simulink model "basic_dynamic_ant"  (R2022a)
settings: Solver=VariableStepAuto  StartTime=0.0  StopTime=10.0  RelTol=1e-3
values from neighbouring files (symbols this model uses):
  configSequence = [robot.Bodies{4}.Joint.PositionLimits; -robot.Bodies{7}.Joint.PositionLimits]    [ant_grasp_only.m]
  dq0 = zeros(size(q0))    [ant_grasp_only.m]
  q0 = homeConfiguration(robot)    [ant_grasp_only.m]
  widgetDimensions = [0.2 0.02 0.07]    [ant_grasp_only.m]
undefined symbols (not defined in the file or in its folder): CenterTable, Floor, LeftShelf, X, Y, Z
libraries: sm_lib x137, nesl_utility x13, robotmaniplib x3, robotcorelib x1
(part 1 of 5)
settings Model: Creator=eroll  LastModifiedBy=eroll

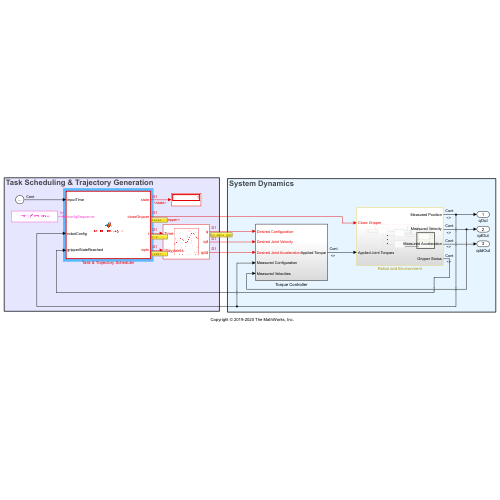
[thumbnail: Simulink's stored preview of the top-level diagram]
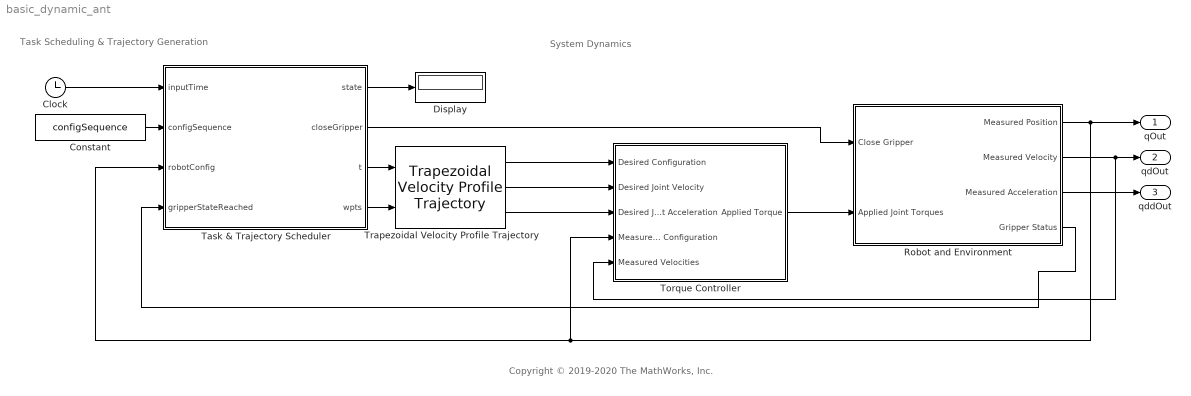
== system basic_dynamic_ant ==
  note: System Dynamics
  note: Copyright © 2019-2020 The MathWorks, Inc.
  note: Task Scheduling & Trajectory Generation
  Clock : Clock
  Constant : Constant  Value=configSequence
  Display : Display
  Robot and Environment : Subsystem
  Task & Trajectory Scheduler : MATLAB Function  TreatAsAtomicUnit=on
  Torque Controller : Subsystem
  Trapezoidal Velocity Profile Trajectory : robotcorelib/Trapezoidal Velocity Profile Trajectory  WaypointSource=External  Waypoints=[ 0, -0.5, -1; 0, 0.5, 1 ]  NumParams=1  Parameter1=End Time  Parameter2=End Time  ParameterSource=Internal  PeakVelocity=[ 2; 2 ]  Acceleration=[ 1; 2 ]  EndTime=2  AccelTime=[ 1; 2 ]  SimulateUsing=Interpreted execution
      settings: SourceProductBaseCode=RO,NV,RR,UV
  qOut : Outport
  qdOut : Outport  Port=2
  qddOut : Outport  Port=3
  wires:
  Task & Trajectory Scheduler/1(state) -> Display/1
  Robot and Environment/4(Gripper Status) -> Task & Trajectory Scheduler/4(gripperStateReached)
  Trapezoidal Velocity Profile Trajectory/1 -> Torque Controller/1(Desired Configuration)
  Clock/1 -> Task & Trajectory Scheduler/1(inputTime)
  Trapezoidal Velocity Profile Trajectory/3 -> Torque Controller/3(Desired Joint Acceleration)
  Trapezoidal Velocity Profile Trajectory/2 -> Torque Controller/2(Desired Joint Velocity)
  Task & Trajectory Scheduler/3(t) -> Trapezoidal Velocity Profile Trajectory/1
  Task & Trajectory Scheduler/4(wpts) -> Trapezoidal Velocity Profile Trajectory/2
  Constant/1 -> Task & Trajectory Scheduler/2(configSequence)
  Task & Trajectory Scheduler/2(closeGripper) -> Robot and Environment/1(Close Gripper)
  Robot and Environment/1(Measured Position) -> Torque Controller/4(Measured Configuration), Task & Trajectory Scheduler/3(robotConfig), qOut/1
  Torque Controller/1(Applied Torque) -> Robot and Environment/2(Applied Joint Torques)
  Robot and Environment/2(Measured Velocity) -> Torque Controller/5(Measured Velocities), qdOut/1
  Robot and Environment/3(Measured Acceleration) -> qddOut/1

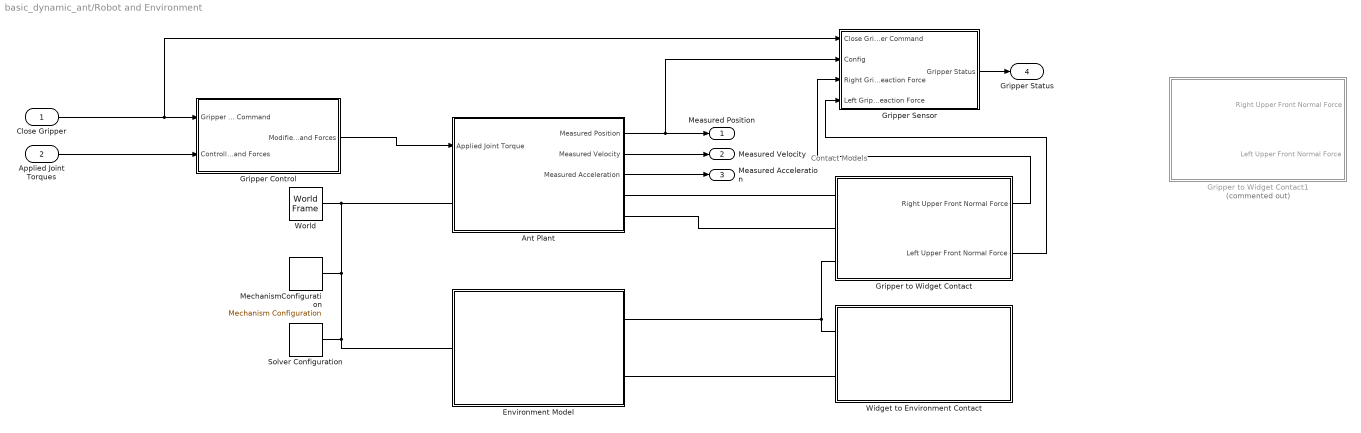
== system basic_dynamic_ant/Robot and Environment ==
  note: Contact Models
  Close Gripper : Inport
  Applied Joint Torques : Inport  Port=2
  Ant Plant : Subsystem
  Environment Model : Subsystem
  Gripper Control : Subsystem
  Gripper Sensor : Subsystem
  Gripper to Widget Contact : Subsystem
  Gripper to Widget Contact1 : Subsystem  Commented=on
  MechanismConfiguration : sm_lib/Utilities/Mechanism Configuration  UniformGravity=Constant  GravityVector=[0 0 -9.80665]  GravityUnits=m/s^2  LinearizationDelta=0.001  JointModeTransitionNonlinearIterations=2
  Solver Configuration : nesl_utility/Solver Configuration  PhysicalDomain=network_engine_domain  SubClassName=solver  LeftPortType=input  RightPortType=generic  Tones=[]  Harmonics=[]  SimulateNoise=off  Profile=off  UseLocalSampling=off  EnableSwitchedLinearOptims=on  FrequencyDomain=off  UseCCode=off  RelTol=0.001  AbsTol=1e-06  MinStep=1e-09  ToWorkspace=off  RevertToSquareIcSolve=off  NumHomotopyIterations=100  PhasorMode=off  PhasorModeNumHarmonics=1  IndexReductionMethod=DerivativeReplacement  DoDC=off  ResidualTolerance=1e-09  UseLocalSolver=off  LocalSolverChoice=NE_BACKWARD_EULER_ADVANCER  LocalSolverSampleTime=0.001  DoFixedCost=off  MaxNonlinIter=3  MaxModeIter=2  ComputeImpulses=off  ImpulseIterations=2  LinearAlgebra=auto  LinearAlgebraNumThread=0  EquationFormulation=NE_TIME_EF  DelaysMemoryBudget=1024  AutomaticFiltering=on  FilteringTimeConstant=0.001  PartitionStorageMethod=AS_NEEDED  PartitionMemoryBudget=1024  PartitionMethod=ROBUST
      settings: SourceProductBaseCode=SS,PW,VE
  Widget to Environment Contact : Subsystem
  World : sm_lib/Frames and Transforms/World Frame
  Measured Position : Outport
  Measured Velocity : Outport  Port=2
  Measured Acceleration : Outport  Port=3
  Gripper Status : Outport  Port=4
  wires:
  Ant Plant/2(Measured Velocity) -> Measured Velocity/1
  Ant Plant/3(Measured Acceleration) -> Measured Acceleration/1
  Applied Joint Torques/1 -> Gripper Control/2(Controller Joint Torques and Forces)
  Gripper Control/1(Modified Joint Torques and Forces) -> Ant Plant/1(Applied Joint Torque)
  Close Gripper/1 -> Gripper Sensor/1(Close Gripper Command), Gripper Control/1(Gripper Close Command)
  Gripper to Widget Contact/1(Right Upper Front Normal Force) -> Gripper Sensor/3(Right Gripper Reaction Force)
  Gripper Sensor/1(Gripper Status) -> Gripper Status/1
  Ant Plant/1(Measured Position) -> Gripper Sensor/2(Config), Measured Position/1
  Gripper to Widget Contact/2(Left Upper Front Normal Force) -> Gripper Sensor/4(Left Gripper Reaction Force)
  connections:
  World/RConn1 -- Ant Plant/LConn1 -- Environment Model/LConn1 -- Solver Configuration/RConn1 -- MechanismConfiguration/RConn1
  Widget to Environment Contact/LConn1 -- Gripper to Widget Contact/LConn3 -- Environment Model/RConn1
  Environment Model/RConn2 -- Widget to Environment Contact/LConn2
  Ant Plant/RConn2 -- Gripper to Widget Contact/LConn2
  Ant Plant/RConn1 -- Gripper to Widget Contact/LConn1

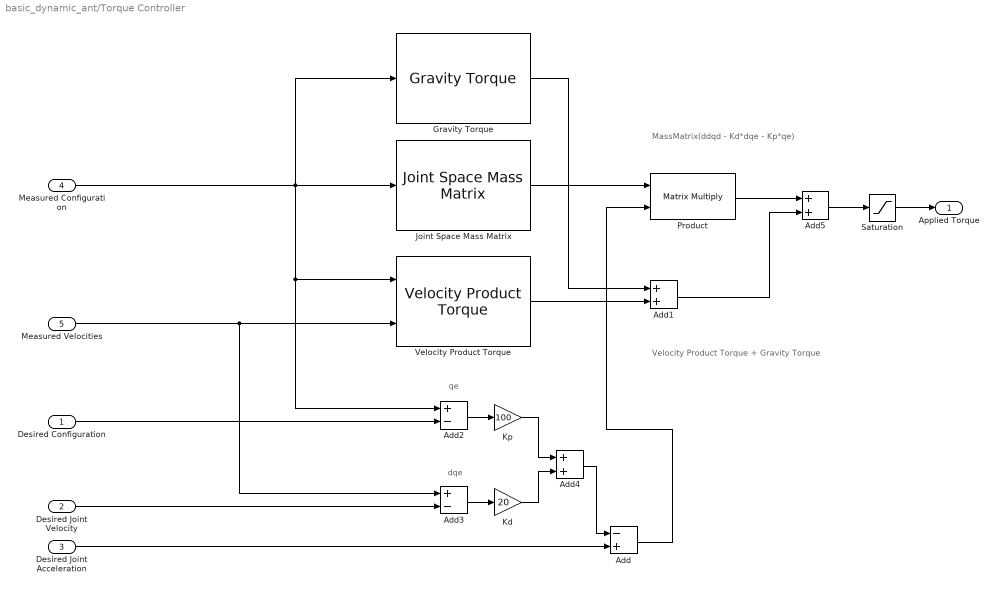
== system basic_dynamic_ant/Torque Controller ==
  note: qe
  note: dqe
  note: Velocity Product Torque + Gravity Torque
  note: MassMatrix(ddqd - Kd*dqe - Kp*qe)
  Desired Configuration : Inport
  Desired Joint Velocity : Inport  Port=2
  Desired Joint Acceleration : Inport  Port=3
  Measured Configuration : Inport  Port=4
  Measured Velocities : Inport  Port=5
  Add : Sum  Inputs=-+
  Add1 : Sum
  Add2 : Sum  Inputs=+-
  Add3 : Sum  Inputs=+-
  Add4 : Sum
  Add5 : Sum
  Gravity Torque : robotmaniplib/Gravity Torque  RigidBodyTree=robot  SimulateUsing=Interpreted execution
  Joint Space Mass Matrix : robotmaniplib/Joint Space Mass Matrix  RigidBodyTree=robot  SimulateUsing=Interpreted execution
  Kd : Gain  Gain=20
  Kp : Gain  Gain=100
  Product : Product  Multiplication=Matrix(*)
  Saturation : Saturate  UpperLimit=100  LowerLimit=-100
  Velocity Product Torque : robotmaniplib/Velocity Product Torque  RigidBodyTree=robot  SimulateUsing=Interpreted execution
      settings: SourceProductBaseCode=RO
  Applied Torque : Outport  VectorParamsAs1DForOutWhenUnconnected=off
  wires:
  Desired Joint Acceleration/1 -> Add/2
  Desired Joint Velocity/1 -> Add3/2
  Desired Configuration/1 -> Add2/2
  Joint Space Mass Matrix/1 -> Product/1
  Measured Configuration/1 -> Joint Space Mass Matrix/1, Gravity Torque/1, Velocity Product Torque/1, Add2/1
  Measured Velocities/1 -> Add3/1, Velocity Product Torque/2
  Add4/1 -> Add/1
  Add/1 -> Product/2
  Add2/1 -> Kp/1
  Add3/1 -> Kd/1
  Kp/1 -> Add4/1
  Kd/1 -> Add4/2
  Add5/1 -> Saturation/1
  Product/1 -> Add5/1
  Add1/1 -> Add5/2
  Gravity Torque/1 -> Add1/1
  Velocity Product Torque/1 -> Add1/2
  Saturation/1 -> Applied Torque/1

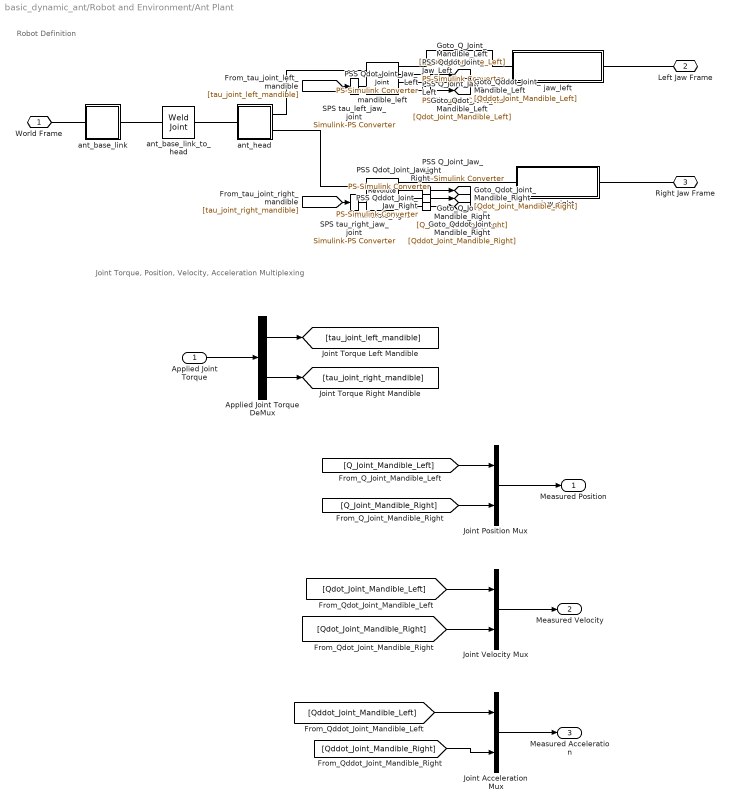
== system basic_dynamic_ant/Robot and Environment/Ant Plant ==
  note: Robot Definition
  note: Joint Torque, Position, Velocity, Acceleration Multiplexing
  Applied Joint Torque : Inport
  Applied Joint Torque DeMux : Demux  Outputs=2
  Joint Acceleration Mux : Mux  Inputs=2
  Joint Position Mux : Mux  Inputs=2
  Joint Velocity Mux : Mux  Inputs=2
  PSS Q_Joint_Jaw_Left : nesl_utility/PS-Simulink Converter  PhysicalDomain=network_engine_domain  SubClassName=ps_output  LeftPortType=input  RightPortType=output  PseudoPeriodic=off  Frequencies=[]  VectorFormat=1-D array  Unit=inherit  AffineConversion=off
      settings: SourceProductBaseCode=SS,PW,VE
  PSS Q_Joint_Jaw_Right : nesl_utility/PS-Simulink Converter  PhysicalDomain=network_engine_domain  SubClassName=ps_output  LeftPortType=input  RightPortType=output  PseudoPeriodic=off  Frequencies=[]  VectorFormat=1-D array  Unit=inherit  AffineConversion=off
      settings: SourceProductBaseCode=SS,PW,VE
  PSS Qddot_Joint_Jaw_Left : nesl_utility/PS-Simulink Converter  PhysicalDomain=network_engine_domain  SubClassName=ps_output  LeftPortType=input  RightPortType=output  PseudoPeriodic=off  Frequencies=[]  VectorFormat=1-D array  Unit=inherit  AffineConversion=off
      settings: SourceProductBaseCode=SS,PW,VE
  PSS Qddot_Joint_Jaw_Right : nesl_utility/PS-Simulink Converter  PhysicalDomain=network_engine_domain  SubClassName=ps_output  LeftPortType=input  RightPortType=output  PseudoPeriodic=off  Frequencies=[]  VectorFormat=1-D array  Unit=inherit  AffineConversion=off
      settings: SourceProductBaseCode=SS,PW,VE
  PSS Qdot_Joint_Jaw_Left : nesl_utility/PS-Simulink Converter  PhysicalDomain=network_engine_domain  SubClassName=ps_output  LeftPortType=input  RightPortType=output  PseudoPeriodic=off  Frequencies=[]  VectorFormat=1-D array  Unit=inherit  AffineConversion=off
      settings: SourceProductBaseCode=SS,PW,VE
  PSS Qdot_Joint_Jaw_Right : nesl_utility/PS-Simulink Converter  PhysicalDomain=network_engine_domain  SubClassName=ps_output  LeftPortType=input  RightPortType=output  PseudoPeriodic=off  Frequencies=[]  VectorFormat=1-D array  Unit=inherit  AffineConversion=off
      settings: SourceProductBaseCode=SS,PW,VE
  SPS tau_left_jaw_joint : nesl_utility/Simulink-PS Converter  PhysicalDomain=network_engine_domain  SubClassName=ps_input  LeftPortType=input  RightPortType=output  PseudoPeriodic=off  Frequencies=[]  NoiseDistribution=none  NoiseParameters=[]  Unit=1  AffineConversion=off  FilteringAndDerivatives=provide  SimscapeFilterOrder=1  InputFilterTimeConstant=0.001  UdotUserProvided=0
      settings: SourceProductBaseCode=SS,PW,VE
  SPS tau_right_jaw_joint : nesl_utility/Simulink-PS Converter  PhysicalDomain=network_engine_domain  SubClassName=ps_input  LeftPortType=input  RightPortType=output  PseudoPeriodic=off  Frequencies=[]  NoiseDistribution=none  NoiseParameters=[]  Unit=1  AffineConversion=off  FilteringAndDerivatives=provide  SimscapeFilterOrder=1  InputFilterTimeConstant=0.001  UdotUserProvided=0
      settings: SourceProductBaseCode=SS,PW,VE
  ant_base_link : Subsystem
  ant_base_link_to_head : sm_lib/Joints/Weld Joint  JointMode=Normal  SenseConstraintForce=off  SenseConstraintForceX=off  SenseConstraintForceY=off  SenseConstraintForceZ=off  SenseConstraintTorque=off  SenseConstraintTorqueX=off  SenseConstraintTorqueY=off  SenseConstraintTorqueZ=off  SenseTotalForce=off  SenseTotalForceX=off  SenseTotalForceY=off  SenseTotalForceZ=off  SenseTotalTorque=off  SenseTotalTorqueX=off  SenseTotalTorqueY=off  SenseTotalTorqueZ=off  CompositeWrenchDir=FollowerOnBase  CompositeWrenchFrame=BaseFrame
  ant_head : Subsystem
  jaw_left : Subsystem
  jaw_right : Subsystem
  mandible_left : sm_lib/Joints/Revolute Joint  JointMode=Normal  SenseConstraintForce=off  SenseConstraintForceX=off  SenseConstraintForceY=off  SenseConstraintForceZ=off  SenseConstraintTorque=off  SenseConstraintTorqueX=off  SenseConstraintTorqueY=off  SenseConstraintTorqueZ=off  SenseTotalForce=off  SenseTotalForceX=off  SenseTotalForceY=off  SenseTotalForceZ=off  SenseTotalTorque=off  SenseTotalTorqueX=off  SenseTotalTorqueY=off  SenseTotalTorqueZ=off  CompositeWrenchDir=FollowerOnBase  CompositeWrenchFrame=BaseFrame  EquilibriumPosition=0  EquilibriumPositionUnits=deg  SpringStiffness=0  SpringStiffnessUnits=N*m/deg  DampingCoefficient=0.5  DampingCoefficientUnits=m^2*kg/s/rad  TorqueActuationMode=InputTorque  MotionActuationMode=ComputedMotion  SensePosition=on  SenseVelocity=on  SenseAcceleration=on  SenseTorqueForce=off  SenseLowerLimitTorqueForce=off  SenseUpperLimitTorqueForce=off  LowerLimitSpecify=on  LowerLimitBound=-2.94087978961  LowerLimitBoundUnits=rad  LowerLimitStiffness=1e4  LowerLimitStiffnessUnits=N*m/deg  LowerLimitDamping=10  LowerLimitDampingUnits=N*m/(deg/s)  LowerLimitTransitionRegionWidth=0.1  LowerLimitTransitionRegionWidthUnits=deg  UpperLimitSpecify=on  UpperLimitBound=2.94087978961  UpperLimitBoundUnits=rad  UpperLimitStiffness=1e4  UpperLimitStiffnessUnits=N*m/deg  UpperLimitDamping=10  UpperLimitDampingUnits=N*m/(deg/s)  UpperLimitTransitionRegionWidth=0.1  UpperLimitTransitionRegionWidthUnits=deg  PositionTargetSpecify=on  PositionTargetPriority=High  PositionTargetValue=q0(1)  PositionTargetValueUnits=rad  VelocityTargetSpecify=on  VelocityTargetPriority=High  VelocityTargetValue=dq0(1)  VelocityTargetValueUnits=rad/s
  mandible_right : sm_lib/Joints/Revolute Joint  JointMode=Normal  SenseConstraintForce=off  SenseConstraintForceX=off  SenseConstraintForceY=off  SenseConstraintForceZ=off  SenseConstraintTorque=off  SenseConstraintTorqueX=off  SenseConstraintTorqueY=off  SenseConstraintTorqueZ=off  SenseTotalForce=off  SenseTotalForceX=off  SenseTotalForceY=off  SenseTotalForceZ=off  SenseTotalTorque=off  SenseTotalTorqueX=off  SenseTotalTorqueY=off  SenseTotalTorqueZ=off  CompositeWrenchDir=FollowerOnBase  CompositeWrenchFrame=BaseFrame  EquilibriumPosition=0  EquilibriumPositionUnits=deg  SpringStiffness=0  SpringStiffnessUnits=N*m/deg  DampingCoefficient=0.5  DampingCoefficientUnits=m^2*kg/s/rad  TorqueActuationMode=InputTorque  MotionActuationMode=ComputedMotion  SensePosition=on  SenseVelocity=on  SenseAcceleration=on  SenseTorqueForce=off  SenseLowerLimitTorqueForce=off  SenseUpperLimitTorqueForce=off  LowerLimitSpecify=off  LowerLimitBound=-2.94087978961  LowerLimitBoundUnits=rad  LowerLimitStiffness=1e4  LowerLimitStiffnessUnits=N*m/deg  LowerLimitDamping=10  LowerLimitDampingUnits=N*m/(deg/s)  LowerLimitTransitionRegionWidth=0.1  LowerLimitTransitionRegionWidthUnits=deg  UpperLimitSpecify=off  UpperLimitBound=2.94087978961  UpperLimitBoundUnits=rad  UpperLimitStiffness=1e4  UpperLimitStiffnessUnits=N*m/deg  UpperLimitDamping=10  UpperLimitDampingUnits=N*m/(deg/s)  UpperLimitTransitionRegionWidth=0.1  UpperLimitTransitionRegionWidthUnits=deg  PositionTargetSpecify=on  PositionTargetPriority=High  PositionTargetValue=q0(2)  PositionTargetValueUnits=rad  VelocityTargetSpecify=on  VelocityTargetPriority=High  VelocityTargetValue=dq0(2)  VelocityTargetValueUnits=rad/s
  World Frame : PMIOPort  Side=Left
  Left Jaw Frame : PMIOPort  Port=2  Side=Right
  Right Jaw Frame : PMIOPort  Port=3  Side=Right
  Measured Position : Outport
  Measured Velocity : Outport  Port=2
  Measured Acceleration : Outport  Port=3
  wires:
  Applied Joint Torque/1 -> Applied Joint Torque DeMux/1
  Applied Joint Torque DeMux/1 -> [tau_joint_left_mandible]
  PSS Qdot_Joint_Jaw_Left/1 -> [Qdot_Joint_Mandible_Left]
  PSS Qdot_Joint_Jaw_Right/1 -> [Qdot_Joint_Mandible_Right]
  PSS Q_Joint_Jaw_Right/1 -> [Q_Joint_Mandible_Right]
  PSS Qddot_Joint_Jaw_Left/1 -> [Qddot_Joint_Mandible_Left]
  PSS Q_Joint_Jaw_Left/1 -> [Q_Joint_Mandible_Left]
  PSS Qddot_Joint_Jaw_Right/1 -> [Qddot_Joint_Mandible_Right]
  [tau_joint_right_mandible] -> SPS tau_right_jaw_joint/1
  [tau_joint_left_mandible] -> SPS tau_left_jaw_joint/1
  Applied Joint Torque DeMux/2 -> [tau_joint_right_mandible]
  [Q_Joint_Mandible_Right] -> Joint Position Mux/2
  [Q_Joint_Mandible_Left] -> Joint Position Mux/1
  Joint Position Mux/1 -> Measured Position/1
  Joint Velocity Mux/1 -> Measured Velocity/1
  [Qdot_Joint_Mandible_Right] -> Joint Velocity Mux/2
  Joint Acceleration Mux/1 -> Measured Acceleration/1
  [Qddot_Joint_Mandible_Right] -> Joint Acceleration Mux/2
  [Qddot_Joint_Mandible_Left] -> Joint Acceleration Mux/1
  [Qdot_Joint_Mandible_Left] -> Joint Velocity Mux/1
  connections:
  mandible_left/LConn2 -- SPS tau_left_jaw_joint/RConn1
  mandible_left/RConn2 -- PSS Q_Joint_Jaw_Left/LConn1
  mandible_left/RConn3 -- PSS Qdot_Joint_Jaw_Left/LConn1
  mandible_right/RConn1 -- jaw_right/LConn1
  mandible_left/RConn1 -- jaw_left/LConn1
  mandible_right/RConn3 -- PSS Qdot_Joint_Jaw_Right/LConn1
  Left Jaw Frame/RConn1 -- jaw_left/RConn1
  mandible_right/RConn2 -- PSS Q_Joint_Jaw_Right/LConn1
  mandible_right/RConn4 -- PSS Qddot_Joint_Jaw_Right/LConn1
  mandible_right/LConn2 -- SPS tau_right_jaw_joint/RConn1
  Right Jaw Frame/RConn1 -- jaw_right/RConn1
  mandible_left/RConn4 -- PSS Qddot_Joint_Jaw_Left/LConn1
  ant_head/RConn2 -- mandible_right/LConn1
  World Frame/RConn1 -- ant_base_link/LConn1
  ant_base_link/RConn1 -- ant_base_link_to_head/LConn1
  ant_head/RConn1 -- mandible_left/LConn1
  ant_head/LConn1 -- ant_base_link_to_head/RConn1

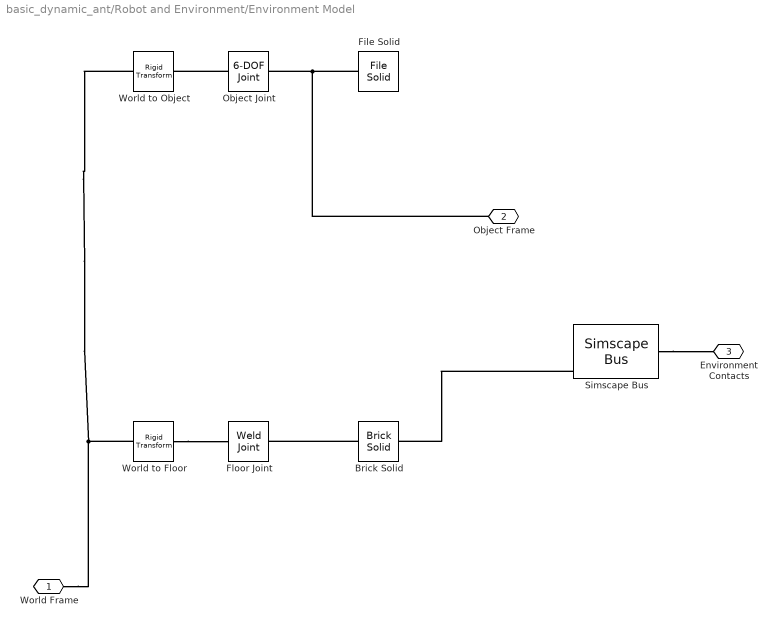
== system basic_dynamic_ant/Robot and Environment/Environment Model ==
  Brick Solid : sm_lib/Body Elements/Brick Solid  GraphicAmbientColor=[0.15 0.15 0.15 1.0]  BasedOnType=Density  BrickDimensions=[20 20 1]  BrickDimensionUnits=cm  CenterOfMass=[0 0 0]  CenterOfMassUnits=m  GraphicDiffuseColor=[0.5 0.5 0.5]  Density=1000  DensityUnits=kg/m^3  DoExposeReferenceFrame=on  GraphicEmissiveColor=[0.0 0.0 0.0 1.0]  ExportEntireGeometry=on  SerializedFrames=<Frames/>  MarkerShape=Sphere  MarkerSize=10  GraphicType=FromGeometry  InertiaType=CalculateFromGeometry  Mass=1  MassUnits=kg  MomentsOfInertia=[1 1 1]  MomentsOfInertiaUnits=kg*m^2  GraphicOpacity=0.2  ProductsOfInertia=[0 0 0]  ProductsOfInertiaUnits=kg*m^2  GraphicShininess=75  GraphicSpecularColor=[0.5 0.5 0.5 1.0]  GraphicVisPropType=SimpleVisualProperties
  File Solid : sm_lib/Body Elements/File Solid  ExtGeomFileName=C:\Users\eroll\Documents\MATLAB\Model\ant_grasp_matlab\AntModel\Environment\Wedge v1.stl  UnitType=Custom  ExtGeomFileUnits=mm  StepReaderType=HEX  ExportConvexHullGeometry=off  InertiaType=CalculateFromGeometry  Mass=1  MassUnits=kg  CenterOfMass=[0 0 0]  CenterOfMassUnits=m  MomentsOfInertia=[1 1 1]  MomentsOfInertiaUnits=kg*m^2  ProductsOfInertia=[0 0 0]  ProductsOfInertiaUnits=kg*m^2  BasedOnType=Density  Density=1000  DensityUnits=kg/m^3  DoExposeReferenceFrame=on  SerializedFrames=<Frames/>  GraphicType=FromGeometry  MarkerShape=Sphere  MarkerSize=10  GraphicVisPropType=SimpleVisualProperties  GraphicDiffuseColor=[0.5 0.5 0.5]  GraphicSpecularColor=[0.5 0.5 0.5 1.0]  GraphicAmbientColor=[0.15 0.15 0.15 1.0]  GraphicEmissiveColor=[0.0 0.0 0.0 1.0]  GraphicShininess=75  GraphicOpacity=1.0
  Floor Joint : sm_lib/Joints/Weld Joint  JointMode=Normal  SenseConstraintForce=off  SenseConstraintForceX=off  SenseConstraintForceY=off  SenseConstraintForceZ=off  SenseConstraintTorque=off  SenseConstraintTorqueX=off  SenseConstraintTorqueY=off  SenseConstraintTorqueZ=off  SenseTotalForce=off  SenseTotalForceX=off  SenseTotalForceY=off  SenseTotalForceZ=off  SenseTotalTorque=off  SenseTotalTorqueX=off  SenseTotalTorqueY=off  SenseTotalTorqueZ=off  CompositeWrenchDir=FollowerOnBase  CompositeWrenchFrame=BaseFrame
  Object Joint : sm_lib/Joints/6-DOF Joint  JointMode=Normal  SenseConstraintForce=off  SenseConstraintForceX=off  SenseConstraintForceY=off  SenseConstraintForceZ=off  SenseConstraintTorque=off  SenseConstraintTorqueX=off  SenseConstraintTorqueY=off  SenseConstraintTorqueZ=off  SenseTotalForce=off  SenseTotalForceX=off  SenseTotalForceY=off  SenseTotalForceZ=off  SenseTotalTorque=off  SenseTotalTorqueX=off  SenseTotalTorqueY=off  SenseTotalTorqueZ=off  CompositeWrenchDir=FollowerOnBase  CompositeWrenchFrame=BaseFrame  PxEquilibriumPosition=0  PxEquilibriumPositionUnits=m  PxSpringStiffness=0  PxSpringStiffnessUnits=N/m  PxDampingCoefficient=0  PxDampingCoefficientUnits=N/(m/s)  PxTorqueActuationMode=NoTorque  PxMotionActuationMode=ComputedMotion  PxSensePosition=off  PxSenseVelocity=off  PxSenseAcceleration=off  PxSenseTorqueForce=off  PxSenseLowerLimitTorqueForce=off  PxSenseUpperLimitTorqueForce=off  PxLowerLimitSpecify=off  PxLowerLimitBound=-1  PxLowerLimitBoundUnits=m  PxLowerLimitStiffness=1e6  PxLowerLimitStiffnessUnits=N/m  PxLowerLimitDamping=1e3  PxLowerLimitDampingUnits=N/(m/s)  PxLowerLimitTransitionRegionWidth=1e-4  PxLowerLimitTransitionRegionWidthUnits=m  PxUpperLimitSpecify=off  PxUpperLimitBound=1  PxUpperLimitBoundUnits=m  PxUpperLimitStiffness=1e6  PxUpperLimitStiffnessUnits=N/m  PxUpperLimitDamping=1e3  PxUpperLimitDampingUnits=N/(m/s)  PxUpperLimitTransitionRegionWidth=1e-4  PxUpperLimitTransitionRegionWidthUnits=m  PxPositionTargetSpecify=off  PxPositionTargetPriority=High  PxPositionTargetValue=0  PxPositionTargetValueUnits=m  PxVelocityTargetSpecify=off  PxVelocityTargetPriority=High  PxVelocityTargetValue=0  PxVelocityTargetValueUnits=m/s  PyEquilibriumPosition=0  PyEquilibriumPositionUnits=m  PySpringStiffness=0  PySpringStiffnessUnits=N/m  PyDampingCoefficient=0  PyDampingCoefficientUnits=N/(m/s)  PyTorqueActuationMode=NoTorque  PyMotionActuationMode=ComputedMotion  PySensePosition=off  PySenseVelocity=off  PySenseAcceleration=off  PySenseTorqueForce=off  PySenseLowerLimitTorqueForce=off  PySenseUpperLimitTorqueForce=off  PyLowerLimitSpecify=off  PyLowerLimitBound=-1  PyLowerLimitBoundUnits=m  PyLowerLimitStiffness=1e6  PyLowerLimitStiffnessUnits=N/m  PyLowerLimitDamping=1e3  PyLowerLimitDampingUnits=N/(m/s)  PyLowerLimitTransitionRegionWidth=1e-4  PyLowerLimitTransitionRegionWidthUnits=m  PyUpperLimitSpecify=off  PyUpperLimitBound=1  PyUpperLimitBoundUnits=m  PyUpperLimitStiffness=1e6  PyUpperLimitStiffnessUnits=N/m  PyUpperLimitDamping=1e3  PyUpperLimitDampingUnits=N/(m/s)  PyUpperLimitTransitionRegionWidth=1e-4  PyUpperLimitTransitionRegionWidthUnits=m  PyPositionTargetSpecify=off  PyPositionTargetPriority=High  PyPositionTargetValue=0  PyPositionTargetValueUnits=m  PyVelocityTargetSpecify=off  PyVelocityTargetPriority=High  PyVelocityTargetValue=0  PyVelocityTargetValueUnits=m/s  PzEquilibriumPosition=0  PzEquilibriumPositionUnits=m  PzSpringStiffness=0  PzSpringStiffnessUnits=N/m  PzDampingCoefficient=0  PzDampingCoefficientUnits=N/(m/s)  PzTorqueActuationMode=NoTorque  PzMotionActuationMode=ComputedMotion  PzSensePosition=off  PzSenseVelocity=off  PzSenseAcceleration=off  PzSenseTorqueForce=off  PzSenseLowerLimitTorqueForce=off  PzSenseUpperLimitTorqueForce=off  PzLowerLimitSpecify=off  PzLowerLimitBound=-1  PzLowerLimitBoundUnits=m  PzLowerLimitStiffness=1e6  PzLowerLimitStiffnessUnits=N/m  PzLowerLimitDamping=1e3  PzLowerLimitDampingUnits=N/(m/s)  PzLowerLimitTransitionRegionWidth=1e-4  PzLowerLimitTransitionRegionWidthUnits=m  PzUpperLimitSpecify=off  PzUpperLimitBound=1  PzUpperLimitBoundUnits=m  PzUpperLimitStiffness=1e6  PzUpperLimitStiffnessUnits=N/m  PzUpperLimitDamping=1e3  PzUpperLimitDampingUnits=N/(m/s)  PzUpperLimitTransitionRegionWidth=1e-4  PzUpperLimitTransitionRegionWidthUnits=m  PzPositionTargetSpecify=on  PzPositionTargetPriority=High  PzPositionTargetValue=0.01  PzPositionTargetValueUnits=m  PzVelocityTargetSpecify=off  PzVelocityTargetPriority=High  PzVelocityTargetValue=0  PzVelocityTargetValueUnits=m/s  SphDefPosRotationMethod=None  SphDefPosRotationAngleUnits=deg  SphDefPosRotationStandardAxis=+Z  SphDefPosRotationAngle=0.0  SphDefPosRotationArbitraryAxis=[0 0 1]  SphDefPosFollAlignAxisA=+X  SphDefPosBaseAlignAxisA=+Y  SphDefPosFollAlignAxisB=+Y  SphDefPosBaseAlignAxisB=+Z  SphDefPosRotationSequenceAxes=FollowerAxes  SphDefPosRotationSequence=XYX  SphDefPosRotationSequenceAngles=[0 0 0]  SphDefPosRotationSequenceAnglesUnits=deg  SphDefPosRotationMatrix=[1 0 0; 0 1 0; 0 0 1]  SphEqPosRotationMethod=None  SphEqPosRotationAngleUnits=deg  SphEqPosRotationStandardAxis=+Z  SphEqPosRotationAngle=0.0  SphEqPosRotationArbitraryAxis=[0 0 1]  SphEqPosFollAlignAxisA=+X  SphEqPosBaseAlignAxisA=+Y  SphEqPosFollAlignAxisB=+Y  SphEqPosBaseAlignAxisB=+Z  SphEqPosRotationSequenceAxes=FollowerAxes  SphEqPosRotationSequence=XYX  SphEqPosRotationSequenceAngles=[0 0 0]  SphEqPosRotationSequenceAnglesUnits=deg  SphEqPosRotationMatrix=[1 0 0; 0 1 0; 0 0 1]  SphSpringStiffness=0  SphSpringStiffnessUnits=N*m/deg  SphDampingCoefficient=0  SphDampingCoefficientUnits=N*m/(deg/s)  SphActuateTorqueX=off  SphActuateTorqueY=off  SphActuateTorqueZ=off  SphActuateTorque=off  SphTorqueActuationMode=NoTorque  SphMotionActuationMode=ComputedMotion  SphActuationFrame=BaseFrame  SphSensePosition=off  SphSenseVelocityX=off  SphSenseVelocityY=off  SphSenseVelocityZ=off  SphSenseVelocity=off  SphSenseAccelerationX=off  SphSenseAccelerationY=off  SphSenseAccelerationZ=off  SphSenseAcceleration=off  SphSenseTorqueX=off  SphSenseTorqueY=off  SphSenseTorqueZ=off  SphSenseTorqueForce=off  SphSenseLowerLimitTorqueMag=off  SphSenseUpperLimitTorqueMag=off  SphSensingFrame=BaseFrame  SphLowerLimitSpecify=off  SphLowerLimitBound=15  SphLowerLimitBoundUnits=deg  SphLowerLimitStiffness=1e4  SphLowerLimitStiffnessUnits=N*m/deg  SphLowerLimitDamping=10  SphLowerLimitDampingUnits=N*m/(deg/s)  SphLowerLimitTransitionRegionWidth=0.1  SphLowerLimitTransitionRegionWidthUnits=deg  SphUpperLimitSpecify=off  SphUpperLimitBound=45  SphUpperLimitBoundUnits=deg  SphUpperLimitStiffness=1e4  SphUpperLimitStiffnessUnits=N*m/deg  SphUpperLimitDamping=10  SphUpperLimitDampingUnits=N*m/(deg/s)  SphUpperLimitTransitionRegionWidth=0.1  SphUpperLimitTransitionRegionWidthUnits=deg  SphPositionTargetRotationMethod=None  SphPositionTargetRotationAngleUnits=deg  SphPositionTargetRotationStandardAxis=+Z  SphPositionTargetRotationAngle=0.0  SphPositionTargetRotationArbitraryAxis=[0 0 1]  SphPositionTargetFollAlignAxisA=+X  SphPositionTargetBaseAlignAxisA=+Y  SphPositionTargetFollAlignAxisB=+Y  SphPositionTargetBaseAlignAxisB=+Z  SphPositionTargetRotationSequenceAxes=FollowerAxes  SphPositionTargetRotationSequence=XYX  SphPositionTargetRotationSequenceAngles=[0 0 0]  SphPositionTargetRotationSequenceAnglesUnits=deg  SphPositionTargetRotationMatrix=[1 0 0; 0 1 0; 0 0 1]  SphPositionTargetSpecify=off  SphPositionTargetPriority=High  SphVelocityTargetValue=[0 0 0]  SphVelocityTargetValueUnits=deg/s  SphVelocityTargetSpecify=off  SphVelocityTargetPriority=High  SphVelocityTargetInFollowerFrame=on
  Simscape Bus : SimscapeBus  HierarchyStrings=CenterTable;LeftShelf;Floor
  World to Floor : sm_lib/Frames and Transforms/Rigid Transform  TranslationMethod=Cartesian  TranslationStandardOffset=0  TranslationLengthUnit=cm  TranslationStandardAxis=+Z  TranslationCartesianOffset=[0, 0, -3]  TranslationROffset=0  TranslationROffsetUnits=m  TranslationZOffset=0  TranslationZOffsetUnits=m  TranslationThetaOffset=0  TranslationThetaOffsetUnits=deg  RotationMethod=None  RotationAngleUnits=deg  RotationStandardAxis=+Z  RotationAngle=0.0  RotationArbitraryAxis=[0 0 1]  FollAlignAxisA=+X  BaseAlignAxisA=+Y  FollAlignAxisB=+Y  BaseAlignAxisB=+Z  RotationSequenceAxes=BaseAxes  RotationSequence=XYZ  RotationSequenceAngles=[0, 0, 0]  RotationSequenceAnglesUnits=rad  RotationMatrix=[1 0 0; 0 1 0; 0 0 1]
  World to Object : sm_lib/Frames and Transforms/Rigid Transform  TranslationMethod=Cartesian  TranslationStandardOffset=0  TranslationLengthUnit=cm  TranslationStandardAxis=+Z  TranslationCartesianOffset=[1, 0, 1]  TranslationROffset=0  TranslationROffsetUnits=m  TranslationZOffset=0  TranslationZOffsetUnits=m  TranslationThetaOffset=0  TranslationThetaOffsetUnits=deg  RotationMethod=None  RotationAngleUnits=deg  RotationStandardAxis=+Z  RotationAngle=0.0  RotationArbitraryAxis=[0 0 1]  FollAlignAxisA=+X  BaseAlignAxisA=+Y  FollAlignAxisB=+Y  BaseAlignAxisB=+Z  RotationSequenceAxes=BaseAxes  RotationSequence=XYZ  RotationSequenceAngles=[0, 0, 0]  RotationSequenceAnglesUnits=rad  RotationMatrix=[1 0 0; 0 1 0; 0 0 1]
  World Frame : PMIOPort  Side=Left
  Object Frame : PMIOPort  Port=2  Side=Right
  Environment Contacts : PMIOPort  Port=3  Side=Right
  connections:
  World to Floor/LConn1 -- World to Object/LConn1 -- World Frame/RConn1
  Simscape Bus/RConn1 -- Environment Contacts/RConn1
  Simscape Bus/LConn3 -- Brick Solid/LConn1
  Brick Solid/RConn1 -- Floor Joint/RConn1
  World to Floor/RConn1 -- Floor Joint/LConn1
  File Solid/RConn1 -- Object Frame/RConn1 -- Object Joint/RConn1
  Object Joint/LConn1 -- World to Object/RConn1

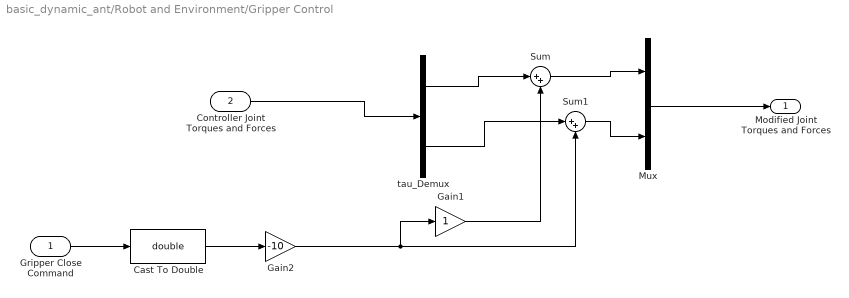
== system basic_dynamic_ant/Robot and Environment/Gripper Control ==
  Gripper Close Command : Inport
  Controller Joint Torques and Forces : Inport  Port=2
  Cast To Double : DataTypeConversion  OutDataTypeStr=double  SaturateOnIntegerOverflow=off  RndMeth=Floor
  Gain1 : Gain
  Gain2 : Gain  Gain=-10
  Mux : Mux  Inputs=2
  Sum : Sum  Inputs=|++
  Sum1 : Sum  Inputs=|++
  tau_Demux : Demux  Outputs=2
  Modified Joint Torques and Forces : Outport
  wires:
  Sum1/1 -> Mux/2
  tau_Demux/1 -> Sum/1
  Gain2/1 -> Sum1/2, Gain1/1
  Gain1/1 -> Sum/2
  Sum/1 -> Mux/1
  Cast To Double/1 -> Gain2/1
  tau_Demux/2 -> Sum1/1
  Controller Joint Torques and Forces/1 -> tau_Demux/1
  Gripper Close Command/1 -> Cast To Double/1
  Mux/1 -> Modified Joint Torques and Forces/1

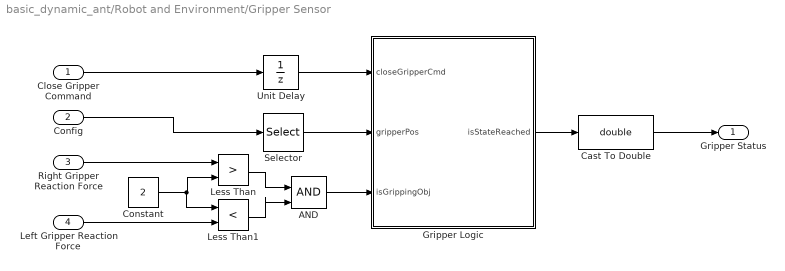
== system basic_dynamic_ant/Robot and Environment/Gripper Sensor ==
  Close Gripper Command : Inport
  Config : Inport  Port=2
  Right Gripper Reaction Force : Inport  Port=3
  Left Gripper Reaction Force : Inport  Port=4
  AND : Logic  IconShape=distinctive  AllPortsSameDT=off  OutDataTypeStr=boolean
  Cast To Double : DataTypeConversion  OutDataTypeStr=double  SaturateOnIntegerOverflow=off  RndMeth=Floor
  Constant : Constant  Value=2
  Gripper Logic : MATLAB Function  TreatAsAtomicUnit=on
  Less Than : RelationalOperator  Operator=>  OutDataTypeStr=boolean  RndMeth=Simplest  InputSameDT=off
  Less Than1 : RelationalOperator  Operator=<  OutDataTypeStr=boolean  RndMeth=Simplest  InputSameDT=off
  Selector : Selector  InputPortWidth=2  IndexOptions=Index vector (dialog)  Indices=[1 2]  OutputSizes=1
  Unit Delay : UnitDelay  SampleTime=-1  HasFrameUpgradeWarning=on
  Gripper Status : Outport
  wires:
  Selector/1 -> Gripper Logic/2(gripperPos)
  Config/1 -> Selector/1
  Constant/1 -> Less Than/2, Less Than1/1
  Unit Delay/1 -> Gripper Logic/1(closeGripperCmd)
  AND/1 -> Gripper Logic/3(isGrippingObj)
  Less Than1/1 -> AND/2
  Gripper Logic/1(isStateReached) -> Cast To Double/1
  Cast To Double/1 -> Gripper Status/1
  Less Than/1 -> AND/1
  Left Gripper Reaction Force/1 -> Less Than1/2
  Right Gripper Reaction Force/1 -> Less Than/1
  Close Gripper Command/1 -> Unit Delay/1
